simulink model "amostraAA3"  (R2021a)
settings: Solver=VariableStepAuto  StartTime=0.0  StopTime=500  RelTol=1e-3
libraries: simulink x1
settings Model: Creator=jhaid  LastModifiedBy=jhaid

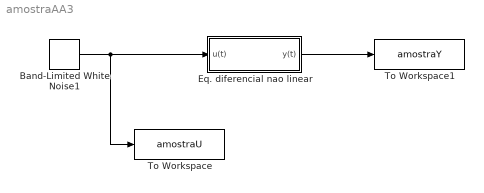
== system amostraAA3 ==
  Band-Limited White Noise1 : simulink/Sources/Band-Limited White Noise  Cov=[1]  Ts=1  seed=[21356]
  Eq. diferencial nao linear : Subsystem
  To Workspace : ToWorkspace  VariableName=amostraU  SaveFormat=Timeseries  SampleTime=-1
  To Workspace1 : ToWorkspace  VariableName=amostraY  SaveFormat=Timeseries  SampleTime=1
  wires:
  Band-Limited White Noise1/1 -> Eq. diferencial nao linear/1(u(t)), To Workspace/1
  Eq. diferencial nao linear/1(y(t)) -> To Workspace1/1

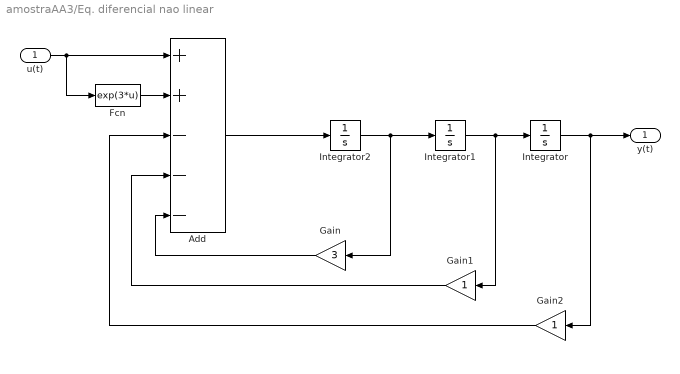
== system amostraAA3/Eq. diferencial nao linear ==
  u(t) : Inport
  Add : Sum  Inputs=++---
  Fcn : Fcn  Expr=exp(3*u)
  Gain : Gain  Gain=3
  Gain1 : Gain
  Gain2 : Gain
  Integrator : Integrator
  Integrator1 : Integrator
  Integrator2 : Integrator
  y(t) : Outport
  wires:
  Add/1 -> Integrator2/1
  Integrator/1 -> y(t)/1, Gain2/1
  Integrator1/1 -> Integrator/1, Gain1/1
  Integrator2/1 -> Integrator1/1, Gain/1
  u(t)/1 -> Fcn/1, Add/1
  Gain/1 -> Add/5
  Gain1/1 -> Add/4
  Gain2/1 -> Add/3
  Fcn/1 -> Add/2
